simulink model "universal_pid"  (R2019a)
settings: Solver=VariableStepAuto  StartTime=0.0  StopTime=10.0  RelTol=1e-3
undefined symbols (not defined in the file or in its folder): b, c, Kp, Td, Tf, Ti
settings Model: Creator=user1  LastModifiedBy=user1

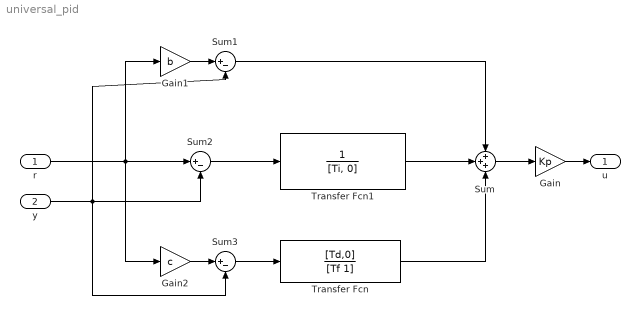
== system universal_pid ==
  "r " : Inport
  y : Inport  Port=2
  Gain : Gain  Gain=Kp
  Gain1 : Gain  Gain=b
  Gain2 : Gain  Gain=c
  Sum : Sum  Inputs=+++
  Sum1 : Sum  Inputs=|+-
  Sum2 : Sum  Inputs=|+-
  Sum3 : Sum  Inputs=|+-
  Transfer Fcn : TransferFcn  Numerator=[Td,0]  Denominator=[Tf 1]
  Transfer Fcn1 : TransferFcn  Denominator=[Ti, 0]
  "u " : Outport
  wires:
  Transfer Fcn1/1 -> Sum/2
  Transfer Fcn/1 -> Sum/3
  Sum/1 -> Gain/1
  Gain1/1 -> Sum1/1
  Sum2/1 -> Transfer Fcn1/1
  Sum1/1 -> Sum/1
  "r "/1 -> Gain2/1, Sum2/1, Gain1/1
  Gain2/1 -> Sum3/1
  y/1 -> Sum2/2, Sum3/2, Sum1/2
  Sum3/1 -> Transfer Fcn/1
  Gain/1 -> "u "/1
